simulink model "torque_model_validation_1"  (R2023b)
settings: Solver=FixedStepAuto  StartTime=0.0  StopTime=32  RelTol=1e-3  EnableMultiTasking=on
libraries: simulink x1
settings Model: SimulationMode=external  ExtModeTrigDuration=10  Creator=kiraa  LastModifiedBy=kiraa
settings SolverCC: InsertRTBMode=Always
settings OptimizationCC: StrengthReduction=on  PassReuseOutputArgsAs=Individual arguments  ZeroExternalMemoryAtStartup=off  ZeroInternalMemoryAtStartup=off  MaxStackSize=64  SimCompilerOptimization=on  OptimizeBlockOrder=speed  OptimizationPriority=Speed  OptimizationCustomize=off  MultiThreadedLoops=on  EfficientTunableParamExpr=on
settings DebuggingCC: ParameterTunabilityLossMsg=error
settings HardwareCC: ProdBitPerPointer=32  ProdBitPerSizeT=32  ProdBitPerPtrDiffT=32  ProdLargestAtomicInteger=Long  ProdLargestAtomicFloat=Double  ProdWordSize=32  ProdLongLongMode=on  ProdHWDeviceType=ARM Compatible->ARM Cortex
settings SFSimCC: MATLABDynamicMemAlloc=off
settings RTWCC: Description=Embedded Coder  SystemTargetFile=ert.tlc  HardwareBoard=STM32 Nucleo F401RE  TemplateMakefile=ert_default_tmf  Toolchain=GNU Tools for ARM Embedded Processors  BuildConfiguration=Faster Runs
settings CodeAppCC: ForceParamTrailComments=on  IgnoreCustomStorageClasses=off  OperatorAnnotations=on  SimulinkDataObjDesc=on  SFDataObjDesc=on  InsertBlockDesc=on
settings ERTTargetCC: CodeReplacementLibrary=ARM Cortex-M  ExtModeTransport=3  ExtModeStaticAlloc=on  ExtModeStaticAllocSize=2000  ExtModeMexFile=ext_xcp  ExtModeIntrfLevel=Level2 - Open

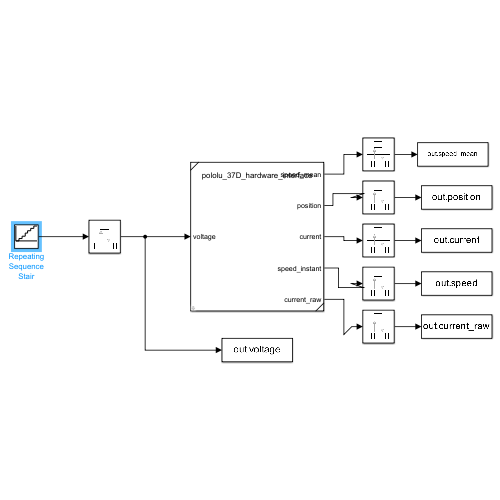
[thumbnail: Simulink's stored preview of the top-level diagram]
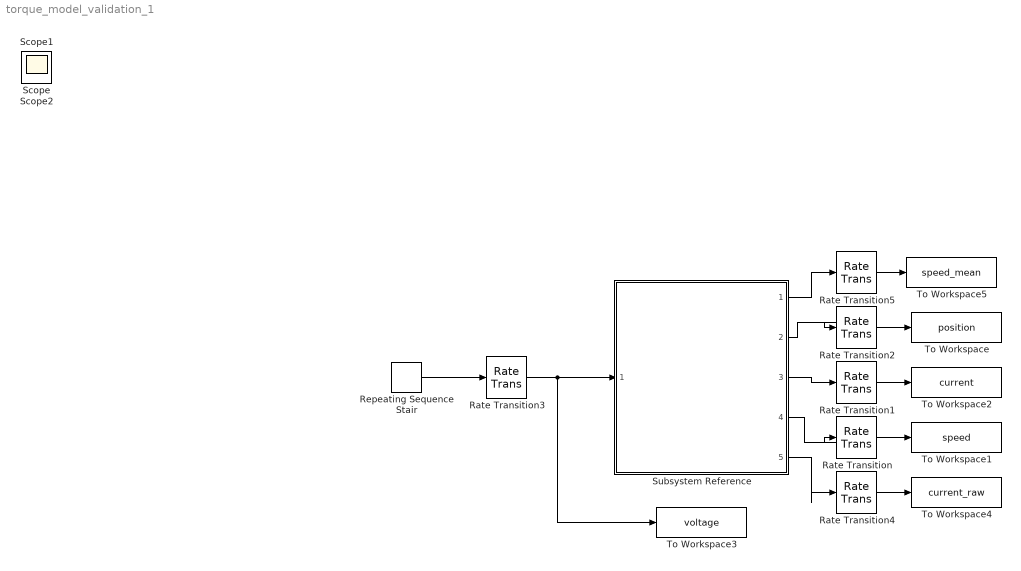
== system torque_model_validation_1 ==
  Rate Transition{,1..5} (6 alike) : RateTransition  OutPortSampleTime=0.005
  Repeating Sequence Stair : simulink/Sources/Repeating Sequence Stair  OutValues=[0:2:12].'  tsamp=4  OutMin=[]  OutMax=[]  OutDataTypeStr=double  OutputDataTypeScalingMode=double  OutDataType=fixdt(0,8)  ConRadixGroup=Best Precision: Vector-wise  OutScaling=2^-12
  Subsystem Reference : Subsystem  ReferencedSubsystem=pololu_37D_hardware_interface  Ts=0.005  pwmFreq=2000
  To Workspace : ToWorkspace  VariableName=position  SaveFormat=Timeseries  SampleTime=-1
  To Workspace1 : ToWorkspace  VariableName=speed  SaveFormat=Timeseries  SampleTime=-1
  To Workspace2 : ToWorkspace  VariableName=current  SaveFormat=Timeseries  SampleTime=-1
  To Workspace3 : ToWorkspace  VariableName=voltage  SaveFormat=Timeseries  SampleTime=-1
  To Workspace4 : ToWorkspace  VariableName=current_raw  SaveFormat=Timeseries  SampleTime=-1
  To Workspace5 : ToWorkspace  VariableName=speed_mean  SaveFormat=Timeseries  SampleTime=-1
  Scope : Scope
  Scope1 : Scope
  Scope2 : Scope
  wires:
  Subsystem Reference/2 -> Rate Transition2/1
  Subsystem Reference/3 -> Rate Transition1/1
  Subsystem Reference/4 -> Rate Transition/1
  Rate Transition/1 -> To Workspace1/1
  Rate Transition1/1 -> To Workspace2/1
  Rate Transition2/1 -> To Workspace/1
  Subsystem Reference/5 -> Rate Transition4/1
  Rate Transition4/1 -> To Workspace4/1
  Subsystem Reference/1 -> Rate Transition5/1
  Rate Transition5/1 -> To Workspace5/1
  Rate Transition3/1 -> To Workspace3/1, Subsystem Reference/1
  Repeating Sequence Stair/1 -> Rate Transition3/1
